simulink model "hw_interrupt"  (R2020b)
settings: Solver=VariableStepAuto  StartTime=0.0  StopTime=10.0  RelTol=1e-3
libraries: arduinolib x1
settings Model: Creator=callum  LastModifiedBy=callum

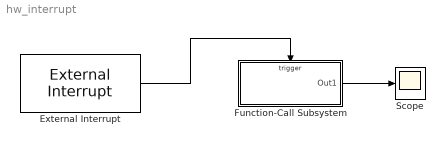
== system hw_interrupt ==
  External Interrupt : arduinolib/External Interrupt  Pin=2  PullUp=off  Mode=RISING  InterruptSimulationInput=off
      settings: SourceProductBaseCode=ARDUINO
  Function-Call Subsystem : Subsystem  TreatAsAtomicUnit=on
  Scope : Scope
  wires:
  External Interrupt/1 -> Function-Call Subsystem/Trigger
  Function-Call Subsystem/1(Out1) -> Scope/1

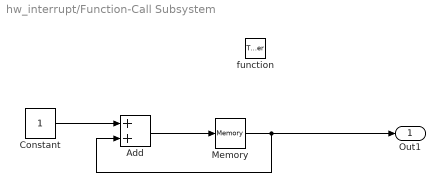
== system hw_interrupt/Function-Call Subsystem ==
  function : TriggerPort  TriggerType=function-call  VariantControl=Variant
  Add : Sum
  Constant : Constant  SampleTime=-1
  Memory : Memory  InheritSampleTime=on
  Out1 : Outport
  wires:
  Memory/1 -> Add/2, Out1/1
  Add/1 -> Memory/1
  Constant/1 -> Add/1
